simulink model "iio_source_sim"  (R2014a)
settings: Solver=ode45  StartTime=0.0  StopTime=Inf  RelTol=1e-3
settings Model: Creator=ACozma  LastModifiedBy=ACozma
settings DebuggingCC: UnderspecifiedInitializationDetection=Classic

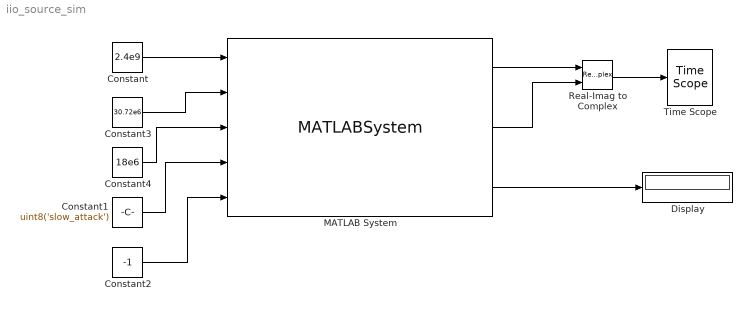
== system iio_source_sim ==
  Constant : Constant  Value=2.4e9
  Constant1 : Constant  Value=uint8('slow_attack')
  Constant2 : Constant  Value=-1
  Constant3 : Constant  Value=30.72e6
  Constant4 : Constant  Value=18e6
  Display : Display
  MATLAB System : MATLABSystem  DialogController=sysobjdialog.BlockDynDialog  System=iio_sys_obj_source  SimulateUsing=Interpreted execution  ip_address=10.50.1.147  dev_name=ad9361  ch_size=32768  ch_no=2
      mask Type: iio_sys_obj_source
      mask Display:
      | disp('ad9361 source');
      | port_label('input',1,'LO_FREQ');
      | port_label('input',2,'SAMPLING_FREQ');
      | port_label('input',3,'RF_BANDWIDTH');
      | port_label('input',4,'RX1_GAIN_MODE');
      | port_label('input',5,'RX1_GAIN');
      | port_label('output',1,'Out1');
      | port_label('output',2,'Out2');
      | port_label('output',3,'RX1_RSSI');
  Real-Imag to Complex : RealImagToComplex  SampleTime=50
  Time Scope : TimeScope  DefaultConfigurationName=spbscopes.TimeScopeBlockCfg
  wires:
  MATLAB System/1 -> Real-Imag to Complex/1
  Real-Imag to Complex/1 -> Time Scope/1
  MATLAB System/2 -> Real-Imag to Complex/2
  Constant/1 -> MATLAB System/1
  Constant2/1 -> MATLAB System/5
  Constant1/1 -> MATLAB System/4
  Constant3/1 -> MATLAB System/2
  Constant4/1 -> MATLAB System/3
  MATLAB System/3 -> Display/1
